simulink model "hw_lqg"  (R2021b)
settings: Solver=VariableStepAuto  StartTime=0.0  StopTime=50  RelTol=1e-3
values from neighbouring files (symbols this model uses):
  A = [ -(delta+sigma)/m1 sigma/m1 -k/m1 k/m1 ... (first row only)    [hw_lqg.m]
  B = [ 0; 1/m2; 0 ; 0 ]    [hw_lqg.m]
  BF = [ B G ]    [hw_lqg.m]
  C = [0 0 1 0 ... (first row only)    [hw_lqg.m]
  DF = zeros(2,5)    [hw_lqg.m]
undefined symbols (not defined in the file or in its folder): K, L
libraries: simulink x6
settings Model: Creator=Manny  LastModifiedBy=User
settings SolverCC: AlgebraicLoopSolver=TrustRegion
settings DebuggingCC: SFMachineParentedDataDiag=warning

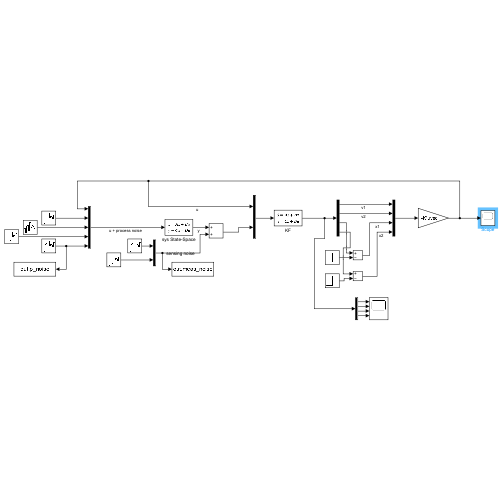
[thumbnail: Simulink's stored preview of the top-level diagram]
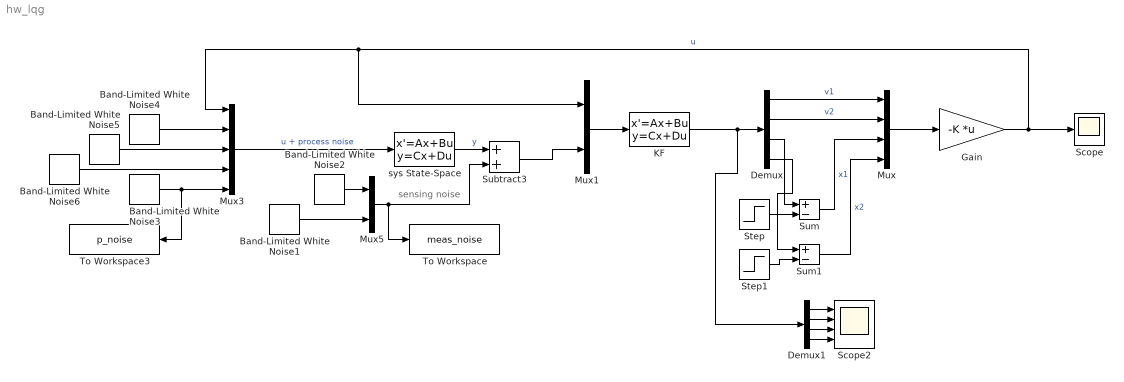
== system hw_lqg ==
  note: sensing noise
  Band-Limited White Noise1 : simulink/Sources/Band-Limited White Noise  Cov=0.000001  Ts=0.01  seed=[23341]
  Band-Limited White Noise{2..6} (5 alike) : simulink/Sources/Band-Limited White Noise  Cov=0.00001  Ts=0.01  seed=[23341]
  Demux : Demux
  Demux1 : Demux
  Gain : Gain  Gain=-K  Multiplication=Matrix(K*u) (u vector)
  KF : StateSpace  A=A-L*C  B=[B L]  C=eye(4)  D=zeros(4,3)  InitialCondition=[0 0 0 0]
  Mux : Mux
  Mux1 : Mux  Inputs=2
  Mux3 : Mux  Inputs=5
  Mux5 : Mux  Inputs=2
  Scope : Scope
  Scope2 : Scope  NumInputPorts=4
  Step : Step  Time=10  After=5  SampleTime=0
  Step1 : Step  Time=10  After=5  SampleTime=0
  Subtract3 : Sum
  Sum : Sum  Inputs=+-
  Sum1 : Sum  Inputs=+-
  To Workspace : ToWorkspace  VariableName=meas_noise  SaveFormat=Timeseries  SampleTime=-1
  To Workspace3 : ToWorkspace  VariableName=p_noise  SaveFormat=Timeseries  SampleTime=-1
  sys State-Space : StateSpace  A=A  B=BF  C=C  D=DF  InitialCondition=[0 0 0 0]
  wires:
  Mux/1 -> Gain/1
  Demux/1 -> Mux/1  "v1"
  Demux/2 -> Mux/2  "v2"
  KF/1 -> Demux1/1, Demux/1
  Step/1 -> Sum/2
  Demux/3 -> Sum/1
  Sum/1 -> Mux/3  "x1"
  Step1/1 -> Sum1/2
  Demux/4 -> Sum1/1
  Sum1/1 -> Mux/4  "x2"
  Demux1/2 -> Scope2/2
  Demux1/1 -> Scope2/1
  Demux1/3 -> Scope2/3
  Demux1/4 -> Scope2/4
  Mux1/1 -> KF/1
  sys State-Space/1 -> Subtract3/1  "y"
  Gain/1 -> Scope/1, Mux1/1, Mux3/1  "u"
  Band-Limited White Noise2/1 -> Mux5/1
  Band-Limited White Noise1/1 -> Mux5/2
  Mux5/1 -> To Workspace/1, Subtract3/2
  Subtract3/1 -> Mux1/2
  Band-Limited White Noise4/1 -> Mux3/2
  Band-Limited White Noise5/1 -> Mux3/3
  Band-Limited White Noise6/1 -> Mux3/4
  Mux3/1 -> sys State-Space/1  "u + process noise"
  Band-Limited White Noise3/1 -> Mux3/5, To Workspace3/1
